simulink model "Erdorbits"  (R2017b)
settings: Solver=VariableStepAuto  StartTime=0.0  StopTime=5532  RelTol=1e-3
settings Model: Creator=aby032  LastModifiedBy=aby032

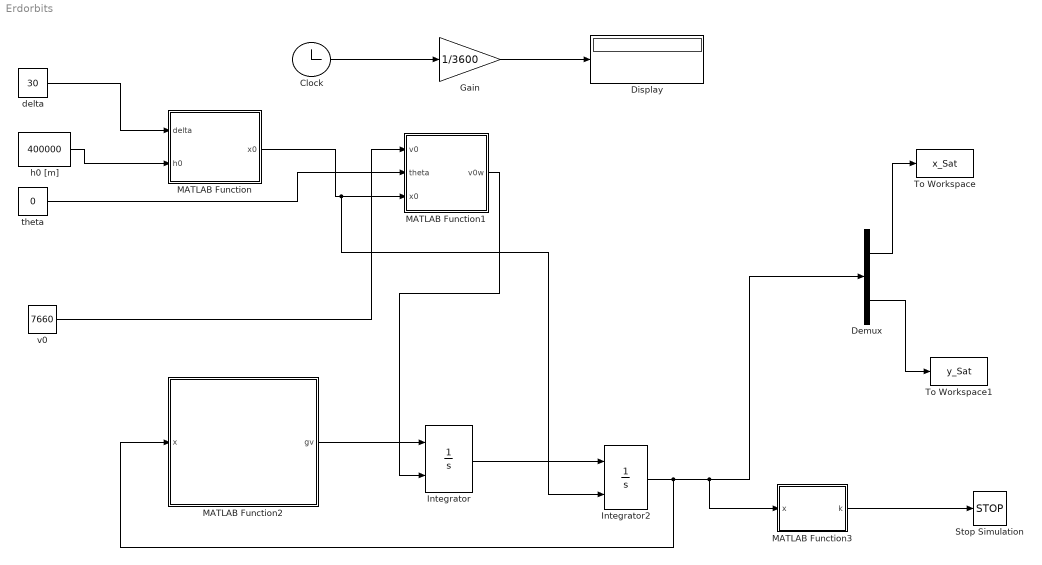
== system Erdorbits ==
  Clock : Clock
      settings: Decimation=2
  Demux : Demux  Outputs=2
  Display : Display
  Gain : Gain  Gain=1/3600
  Integrator : Integrator  InitialConditionSource=external
  Integrator2 : Integrator  InitialConditionSource=external
  MATLAB Function : MATLAB Function  TreatAsAtomicUnit=on
  MATLAB Function1 : MATLAB Function  TreatAsAtomicUnit=on
  MATLAB Function2 : MATLAB Function  TreatAsAtomicUnit=on
  MATLAB Function3 : MATLAB Function  TreatAsAtomicUnit=on
  Stop Simulation : Stop
  To Workspace : ToWorkspace  VariableName=x_Sat  SampleTime=-1
      settings: Save2DSignal=2-D array (concatenate along first dimension)
  To Workspace1 : ToWorkspace  VariableName=y_Sat  SampleTime=-1
      settings: Save2DSignal=2-D array (concatenate along first dimension)
  delta : Constant  Value=30
  h0 [m] : Constant  Value=400000
  theta : Constant  Value=0
  v0 : Constant  Value=7660
  wires:
  Clock/1 -> Gain/1
  Gain/1 -> Display/1
  delta/1 -> MATLAB Function/1(delta)
  h0 [m]/1 -> MATLAB Function/2(h0)
  MATLAB Function/1(x0) -> Integrator2/2, MATLAB Function1/3(x0)
  theta/1 -> MATLAB Function1/2(theta)
  v0/1 -> MATLAB Function1/1(v0)
  MATLAB Function1/1(v0w) -> Integrator/2
  MATLAB Function3/1(k) -> Stop Simulation/1
  Demux/1 -> To Workspace/1
  Demux/2 -> To Workspace1/1
  MATLAB Function2/1(gv) -> Integrator/1
  Integrator/1 -> Integrator2/1
  Integrator2/1 -> MATLAB Function2/1(x), MATLAB Function3/1(x), Demux/1

== matlab function Erdorbits/MATLAB Function1 ==
  data: v0 input; v0w output; theta input; x0 input
function v0w = vStart(v0,theta,x0)
n = x0/norm(x0);
t = [n(2); -n(1)];

vt = cosd(theta)*v0;
vn = sind(theta)*v0;

v0w = vn*n+vt*t;
end

== matlab function Erdorbits/MATLAB Function ==
  data: delta input; x0 output; h0 input
function x0 = Startposition(delta,h0)
re = 6378000; % Erdradius in m

x1 = cosd(delta)*(h0+re)
x2 = sind(delta)*(h0+re)

x0 = [x1; x2]
end

== matlab function Erdorbits/MATLAB Function2 ==
  data: x input; gv output
function gv = Gravitation(x)
G = 66.743e-12      % Gravitationskonstante
me = 5.9736e24      % Masse Erde in kg
xb = norm(x);       % Abstand Erde - Satellit in m
e = x/(-norm(x));   % Einheitsvektor Richtung Satellit -> Erde
gv = G*me/(xb*xb)*e
end

== matlab function Erdorbits/MATLAB Function3 ==
  data: x input; k output
function k = Kontakt(x)
re = 6378000
if re < norm(x)
    k = 0
else
    k = 1
end
